simulink model "secondweektwo"  (R2020a)
settings: Solver=VariableStepAuto  StartTime=0.0  StopTime=10.0  RelTol=1e-3
model workspace (MAT data in the model file):
  Fn = Simulink.Parameter
  Fn.Value = [0  0; 1  0.8; 2  1.6; 3  1.6; 4  1.6; 5  1.6; 6  0.8; 7  0; 8  0; 9  0; 10  0]
  Fn.DataType = 'auto'
  Fn.Dimensions = [11 2]
  R = Simulink.Parameter
  R.Value = 1
  R.DataType = 'auto'
  R.Dimensions = [1 1]
  muk = Simulink.Parameter
  muk.Value = 1
  muk.DataType = 'auto'
  muk.Dimensions = [1 1]
  mus = Simulink.Parameter
  mus.Value = 1.5
  mus.DataType = 'auto'
  mus.Dimensions = [1 1]
settings Model: Creator=Admin  LastModifiedBy=Admin

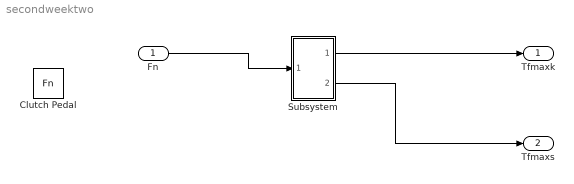
== system secondweektwo ==
  Fn : Inport
  "Clutch Pedal " : Constant  Value=Fn
  Subsystem : Subsystem
  Tfmaxk : Outport
  Tfmaxs : Outport  Port=2
  wires:
  Fn/1 -> Subsystem/1(In1)
  Subsystem/1(Out1) -> Tfmaxk/1
  Subsystem/2(Out2) -> Tfmaxs/1

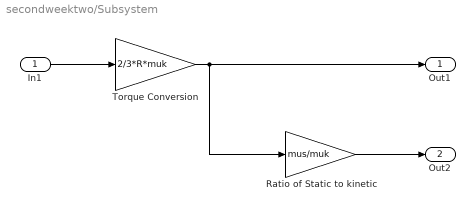
== system secondweektwo/Subsystem ==
  In1 : Inport
  Ratio of Static to kinetic : Gain  Gain=mus/muk
  Torque Conversion : Gain  Gain=2/3*R*muk
  Out1 : Outport
  Out2 : Outport  Port=2
  wires:
  Ratio of Static to kinetic/1 -> Out2/1
  Torque Conversion/1 -> Out1/1, Ratio of Static to kinetic/1
  In1/1 -> Torque Conversion/1
